simulink model "ROKI_3"  (R2016b)
settings: Solver=ode3  StartTime=0.0  StopTime=inf  RelTol=1e-3
libraries: legonxtlib x7, simulink x1
settings Model: SimulationMode=external  ExtModeTrigDuration=2  Creator=The Great Scrublord  LastModifiedBy=Dario Kuvacic
settings DebuggingCC: ParameterTunabilityLossMsg=error
settings HardwareCC: ProdBitPerPointer=32  ProdBitPerSizeT=32  ProdBitPerPtrDiffT=32  ProdLargestAtomicInteger=Long  ProdWordSize=32  ProdHWDeviceType=ARM Compatible->ARM 7
settings RTWCC: SystemTargetFile=realtime.tlc  GenerateMakefile=off  TemplateMakefile=realtime.tmf  Description=Run on Target Hardware  RTWVerbose=off  IncludeHyperlinkInReport=on
settings CodeAppCC: ForceParamTrailComments=on  OperatorAnnotations=on  SimulinkDataObjDesc=on  SFDataObjDesc=on  MATLABFcnDesc=on  InsertBlockDesc=on  MATLABSourceComments=on
settings STFCustomTargetCC: TargetLibSuffix=.a  GenerateSampleERTMain=on  ERTCustomFileBanners=on  SupportNonInlinedSFcns=off  RemoveResetFunc=on  SupportVariableSizeSignals=on  MATLABClassNameForMDSCustomization=Simulink.SoftwareTarget.ERTCustomization  GRTInterface=off  SystemTargetFile=realtime.tlc
settings ERTTargetCC: GenerateSampleERTMain=on  ParMdlRefBuildCompliant=off  CompOptLevelCompliant=off  ConcurrentExecutionCompliant=off  CombineOutputUpdateFcns=off  ERTFirstTimeCompliant=off  SupportContinuousTime=on  SupportVariableSizeSignals=on  ModelStepFunctionPrototypeControlCompliant=off  CPPClassGenCompliant=off  UseToolchainInfoCompliant=off  ExtModeTransport=3  ExtModeMexFile=ext_serial_win32_comm_rtt  ExtModeMexArgs=0 1 9600  ERTSrcFileBannerTemplate=realtime_code_template.cgt  ERTHdrFileBannerTemplate=realtime_code_template.cgt  ERTDataSrcFileTemplate=realtime_code_template.cgt  ERTDataHdrFileTemplate=realtime_code_template.cgt  ERTCustomFileTemplate=realtime_file_process.tlc

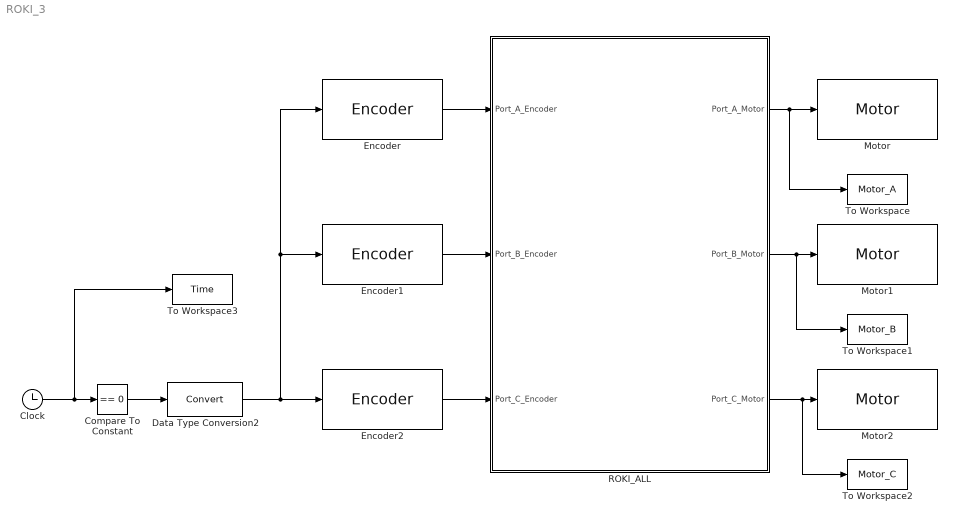
== system ROKI_3 ==
  Clock : Clock
  Compare To Constant : simulink/Logic and Bit Operations/Compare To Constant  relop===  const=0  OutDataTypeStr=boolean
  Data Type Conversion2 : DataTypeConversion
  Encoder : legonxtlib/Encoder  portNumber=A  opMode=Reset by external signal  sampleTime=0.1  blockPlatform=LegoMindstormsNXT
  Encoder1 : legonxtlib/Encoder  portNumber=B  opMode=Reset by external signal  sampleTime=0.1  blockPlatform=LegoMindstormsNXT
  Encoder2 : legonxtlib/Encoder  portNumber=C  opMode=Reset by external signal  sampleTime=0.1  blockPlatform=LegoMindstormsNXT
  Motor : legonxtlib/Motor  sportNumber=A  sstopAction=Brake  blockPlatform=LegoMindstormsNXT
  Motor1 : legonxtlib/Motor  sportNumber=B  sstopAction=Brake  blockPlatform=LegoMindstormsNXT
  Motor2 : legonxtlib/Motor  sportNumber=C  sstopAction=Brake  blockPlatform=LegoMindstormsNXT
  ROKI_ALL : Subsystem
  To Workspace : ToWorkspace  VariableName=Motor_A  SaveFormat=Timeseries  SampleTime=-1
  To Workspace1 : ToWorkspace  VariableName=Motor_B  SaveFormat=Timeseries  SampleTime=-1
  To Workspace2 : ToWorkspace  VariableName=Motor_C  SaveFormat=Timeseries  SampleTime=-1
  To Workspace3 : ToWorkspace  VariableName=Time  SaveFormat=Timeseries  SampleTime=-1
  wires:
  ROKI_ALL/3("Port_C_Motor ") -> To Workspace2/1, Motor2/1
  ROKI_ALL/2(Port_B_Motor) -> To Workspace1/1, Motor1/1
  ROKI_ALL/1(Port_A_Motor) -> To Workspace/1, Motor/1
  Data Type Conversion2/1 -> Encoder/1, Encoder1/1, Encoder2/1
  Clock/1 -> To Workspace3/1, Compare To Constant/1
  Compare To Constant/1 -> Data Type Conversion2/1
  Encoder/1 -> ROKI_ALL/1(Port_A_Encoder)
  Encoder1/1 -> ROKI_ALL/2(Port_B_Encoder)
  Encoder2/1 -> ROKI_ALL/3(Port_C_Encoder)

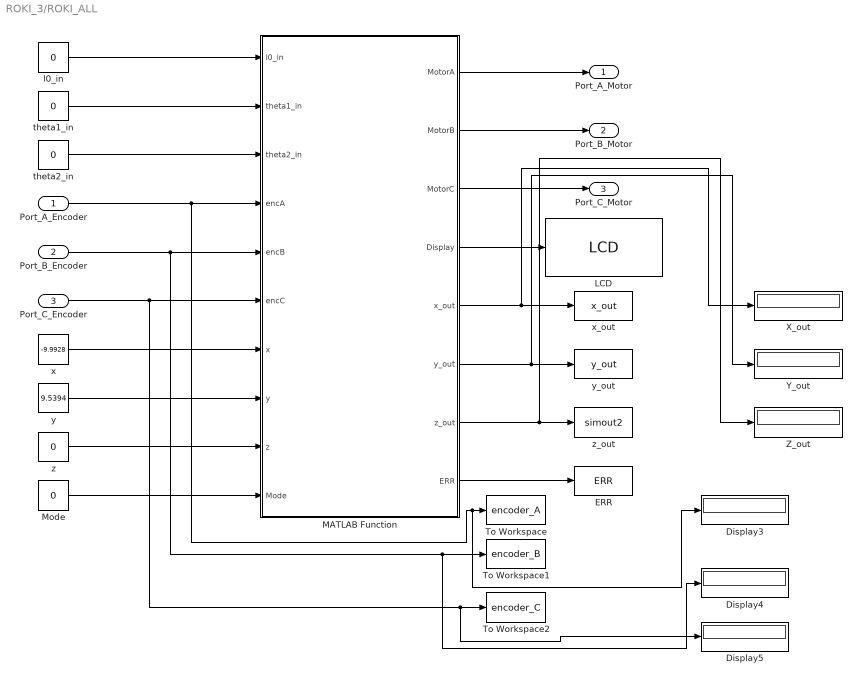
== system ROKI_3/ROKI_ALL ==
  Port_A_Encoder : Inport
  Port_B_Encoder : Inport  Port=2
  Port_C_Encoder : Inport  Port=3
  Display3 : Display
  Display4 : Display
  Display5 : Display
  "ERR " : ToWorkspace  VariableName=ERR  SampleTime=-1
  LCD : legonxtlib/LCD  slcdLine=1  slcdFormat=Decimal  blockPlatform=LegoMindstormsNXT
  MATLAB Function : MATLAB Function  TreatAsAtomicUnit=on
  "Mode " : Constant  Value=0
  To Workspace : ToWorkspace  VariableName=encoder_A  SaveFormat=Timeseries  SampleTime=-1
  To Workspace1 : ToWorkspace  VariableName=encoder_B  SaveFormat=Timeseries  SampleTime=-1
  To Workspace2 : ToWorkspace  VariableName=encoder_C  SaveFormat=Timeseries  SampleTime=-1
  X_out : Display
  Y_out : Display
  Z_out : Display
  "l0_in " : Constant  Value=0
  theta1_in : Constant  Value=0
  theta2_in : Constant  Value=0
  x : Constant  Value=-9.9928
  "x_out " : ToWorkspace  VariableName=x_out  SampleTime=-1
  y : Constant  Value=9.5394
  "y_out " : ToWorkspace  VariableName=y_out  SampleTime=-1
  z : Constant  Value=0
  "z_out " : ToWorkspace  VariableName=simout2  SampleTime=-1
  Port_A_Motor : Outport
  Port_B_Motor : Outport  Port=2
  "Port_C_Motor " : Outport  Port=3
  wires:
  Port_B_Encoder/1 -> Display4/1, To Workspace1/1, MATLAB Function/5(encB)
  Port_A_Encoder/1 -> Display3/1, To Workspace/1, MATLAB Function/4(encA)
  Port_C_Encoder/1 -> Display5/1, To Workspace2/1, MATLAB Function/6(encC)
  MATLAB Function/3(MotorC) -> "Port_C_Motor "/1
  MATLAB Function/2(MotorB) -> Port_B_Motor/1
  MATLAB Function/1(MotorA) -> Port_A_Motor/1
  MATLAB Function/4(Display) -> LCD/1
  x/1 -> MATLAB Function/7(x)
  y/1 -> MATLAB Function/8(y)
  z/1 -> MATLAB Function/9(z)
  theta2_in/1 -> MATLAB Function/3(theta2_in)
  theta1_in/1 -> MATLAB Function/2(theta1_in)
  "l0_in "/1 -> MATLAB Function/1(l0_in)
  MATLAB Function/5(x_out) -> X_out/1, "x_out "/1
  MATLAB Function/6(y_out) -> Y_out/1, "y_out "/1
  MATLAB Function/7(z_out) -> Z_out/1, "z_out "/1
  "Mode "/1 -> MATLAB Function/10(Mode)
  MATLAB Function/8(ERR) -> "ERR "/1

== matlab function ROKI_3/ROKI_ALL/MATLAB Function ==
  data: l0_in input; MotorA output; theta1_in input; theta2_in input; encA input; encB input; encC input; x input; y input; z input; Mode input; MotorB output; MotorC output; Display output; x_out output; y_out output; z_out output; ERR output
function [MotorA, MotorB, MotorC, Display, x_out, y_out, z_out, ERR] = KINEMATIKA(l0_in, theta1_in, theta2_in, encA, encB, encC, x, y, z, Mode)
    encB = encB*(-1);
    encA = encA*(-1);
    MotorA = 0;
    MotorB = 0;
    MotorC = 0;
    a2     = 12.8;
    a3     = 11.3;
    x_out  = 0;
    y_out  = 0;
    z_out  = 0;
    Display = 0;
    l0      = 0;
    theta0  = 0;
    theta1  = 0;
    theta2  = 0;
    ERR = 0;
    neosjetljivost = 3;
    % zracnost_korekcija2 = 14;
    % zracnost_korekcija1 = 8;
    r = 1.15;
    %corr = 0;
    if Mode == 0
    	[l0, theta1, theta2, ERR] = inv_kin(x, y, z, a2, a3);
    else
        l0 = l0_in;
        theta1 = theta1_in/57.295779;
        theta2 = (theta2_in-3/5*theta1_in)/57.295779;
    end
    
    [x_out, y_out, z_out] = dir_kin(encA/(57.295779*r), -1*encB/57.295779, encC/57.295779, a2, a3);
        
    if ERR == 0
        theta0 = l0/r*57.295779;
        theta1 = theta1*57.295779;
        theta2 = theta2*57.295779;

    %     if (theta2 < encC )&& (neosjetljivost*3 < abs(theta2 - encC)) 
    %         theta2 = theta2 - zracnost_korekcija2;
    %     elseif (theta2 > encC)&&(neosjetljivost*3 < abs(theta2 < encC))
    %         theta2 = theta2 + zracnost_korekcija2;
    %     end
    %     if (theta2 < encC )&& (neosjetljivost*2 < abs(theta2 - encC)) 
    %         theta2 = theta2 - 3;
    %     elseif (theta2 > encC)&& (neosjetljivost*2 < abs(theta2 - encC)) 
    %         theta2 = theta2 + 3;
    %     end
    %         
    %     if (theta1 < encB )&& (neosjetljivost+2 < abs(theta1 - encB)) 
    %         theta1 = theta1 - zracnost_korekcija1;
    %         corr = 1;
    %     elseif (theta1 > encB)&&(neosjetljivost+2 < abs(theta1 < encB))
    %         theta1 = theta1 + zracnost_korekcija1;
    %         corr = 1;
    %     end
    %        
    %         theta2 = theta2 + 3/5*zracnost_korekcija1*corr;
    % 
        if theta2<0
            theta2 = theta2-10;
        elseif theta2>0
            theta2 = theta2+10;
        end
        
        if theta1<0
            theta1 = theta1-2;
        elseif theta1>0
            theta1 = theta1+2;
        end    
        

        if(encA < theta0-neosjetljivost-2)||(encA > theta0+neosjetljivost+2) 
            if theta0 > encA
                MotorA = -50;
            else
                MotorA = 25;
            end
        end

        if(encB < theta1-neosjetljivost)||(encB > theta1+neosjetljivost) 
            if theta1 > encB
                MotorB = cast((-15-35*abs(theta2 - encB)/360), 'double');
            else
                MotorB = cast(( 15+35*abs(theta2 - encB)/360), 'double');
            end
        end

        if(encC < theta2-neosjetljivost+1)||(encC > theta2+neosjetljivost-1) 
            if theta2 > encC
                MotorC =  cast(1*( 11+40*abs(theta2 - encC)/360), 'double');

            else
                MotorC = cast(1*(-11-40*abs(theta2 - encC)/360), 'double');

            end

        end
    %else
            %disp('Target out of range - INVERSE.m');
            %Display = 'ERROR';
    end
    
    % disp('MotorA');
    % disp(MotorA);
    % disp('MotorB');
    % disp(MotorB);
    % disp('MotorC');
    % disp(MotorC);
    Display = double(ERR);
    ERR = 10;
end
